simulink model "SPGF_FSK_0000_R2021b"  (R2021b)
settings: Solver=ode4  StartTime=0.0  StopTime=1.4  FixedStep=50e-6/50  RelTol=1e-3  EnableMultiTasking=on
undefined symbols (not defined in the file): D11, Delta
libraries: spsSeriesRLCBranchLib x1645, spsGroundLib x359, spsCurrentMeasurementLib x145, spsIdealSwitchLib x144, spsStairGeneratorLib x135, spsUniversalBridgeLib x76, spsThreePhaseSeriesRLCLoadLib x57, spsSequenceAnalyzerLib x31, simulink x24, spsThreePhaseParallelRLCLoadLib x20, spsThreePhaseTransformerTwoWindingsLib x20, spsDistributedParametersLineLib x19
(part 36 of 36)

== system SPGF_FSK_0000_R2021b/W51/Q/breaker ==
  Fault A2 : Constant  Value=InitialStatus(3)
  Fault A3 : Constant  Value=InitialStatus(2)
  Fault A4 : Constant  Value=InitialStatus(1)
  Fault C1 : Constant  Value=SwitchC
  Fault C2 : Constant  Value=SwitchB
  Fault C3 : Constant  Value=SwitchA
  Ideal Switch A : spsIdealSwitchLib/Ideal Switch  Ron=BreakerResistance  Lon=0  IC=InitialStatus(1)  Rs=SnubberResistance  Cs=SnubberCapacitance  Measurements=off
  Ideal Switch B : spsIdealSwitchLib/Ideal Switch  Ron=BreakerResistance  Lon=0  IC=InitialStatus(2)  Rs=SnubberResistance  Cs=SnubberCapacitance  Measurements=off
  Ideal Switch C : spsIdealSwitchLib/Ideal Switch  Ron=BreakerResistance  Lon=0  IC=InitialStatus(3)  Rs=SnubberResistance  Cs=SnubberCapacitance  Measurements=off
  Stair Generator A : spsStairGeneratorLib/Stair Generator  t=SwitchTimesA  e=SwitchStatusA  Ts=0
  Stair Generator B : spsStairGeneratorLib/Stair Generator  t=SwitchTimesB  e=SwitchStatusB  Ts=0
  Stair Generator C : spsStairGeneratorLib/Stair Generator  t=SwitchTimesC  e=SwitchStatusC  Ts=0
  Switch2 : Switch  Criteria=u2 > Threshold  Threshold=0.5
  Switch3 : Switch  Criteria=u2 > Threshold  Threshold=0.5
  Switch4 : Switch  Criteria=u2 > Threshold  Threshold=0.5
  A : PMIOPort  Side=Left
  B : PMIOPort  Port=2  Side=Left
  C : PMIOPort  Port=3  Side=Left
  a : PMIOPort  Port=4  Side=Right
  b : PMIOPort  Port=5  Side=Right
  c : PMIOPort  Port=6  Side=Right
  wires:
  Switch2/1 -> Ideal Switch C/1
  Fault A2/1 -> Switch2/3
  Fault C1/1 -> Switch2/2
  Switch3/1 -> Ideal Switch B/1
  Fault A3/1 -> Switch3/3
  Fault C2/1 -> Switch3/2
  Fault A4/1 -> Switch4/3
  Fault C3/1 -> Switch4/2
  Switch4/1 -> Ideal Switch A/1
  Stair Generator B/1 -> Switch3/1
  Stair Generator A/1 -> Switch4/1
  Stair Generator C/1 -> Switch2/1
  connections:
  Ideal Switch B/LConn1 -- B/RConn1
  Ideal Switch A/LConn1 -- A/RConn1
  Ideal Switch C/LConn1 -- C/RConn1
  Ideal Switch A/RConn1 -- a/RConn1
  b/RConn1 -- Ideal Switch B/RConn1
  c/RConn1 -- Ideal Switch C/RConn1

== system SPGF_FSK_0000_R2021b/W51/Q/meas ==
  Add : Sum  Inputs=+++
  GainI : Gain
  GainI0 : Gain
  I A: : spsCurrentMeasurementLib/Current Measurement  PhasorSimulation=off  OutputType=Complex  PSBequivalent=0
  I B: : spsCurrentMeasurementLib/Current Measurement  PhasorSimulation=off  OutputType=Complex  PSBequivalent=0
  I C: : spsCurrentMeasurementLib/Current Measurement  PhasorSimulation=off  OutputType=Complex  PSBequivalent=0
  Mux : Mux  Inputs=3
  A : PMIOPort  Side=Left
  B : PMIOPort  Port=2  Side=Left
  C : PMIOPort  Port=3  Side=Left
  a : PMIOPort  Port=4  Side=Right
  b : PMIOPort  Port=5  Side=Right
  c : PMIOPort  Port=6  Side=Right
  tag scope: CT3I0_W51=global, CTIabc_W51=global
  wires:
  I A:/1 -> Mux/1, Add/1
  I B:/1 -> Mux/2, Add/2
  I C:/1 -> Mux/3, Add/3
  Add/1 -> GainI0/1
  GainI0/1 -> [CT3I0_W51]
  Mux/1 -> GainI/1
  GainI/1 -> [CTIabc_W51]
  connections:
  I C:/RConn1 -- c/RConn1
  I B:/RConn1 -- b/RConn1
  a/RConn1 -- I A:/RConn1
  I A:/LConn1 -- A/RConn1
  I C:/LConn1 -- C/RConn1
  I B:/LConn1 -- B/RConn1

== system SPGF_FSK_0000_R2021b/W51/Q/shunt ==
  A : PMIOPort  Side=Left
  B : PMIOPort  Port=2  Side=Left
  C : PMIOPort  Port=3  Side=Left
  a : PMIOPort  Port=4  Side=Right
  b : PMIOPort  Port=5  Side=Right
  c : PMIOPort  Port=6  Side=Right
  connections:
  C/RConn1 -- c/RConn1
  B/RConn1 -- b/RConn1
  A/RConn1 -- a/RConn1

== system SPGF_FSK_0000_R2021b/W52/Q/breaker ==
  Fault A2 : Constant  Value=InitialStatus(3)
  Fault A3 : Constant  Value=InitialStatus(2)
  Fault A4 : Constant  Value=InitialStatus(1)
  Fault C1 : Constant  Value=SwitchC
  Fault C2 : Constant  Value=SwitchB
  Fault C3 : Constant  Value=SwitchA
  Ideal Switch A : spsIdealSwitchLib/Ideal Switch  Ron=BreakerResistance  Lon=0  IC=InitialStatus(1)  Rs=SnubberResistance  Cs=SnubberCapacitance  Measurements=off
  Ideal Switch B : spsIdealSwitchLib/Ideal Switch  Ron=BreakerResistance  Lon=0  IC=InitialStatus(2)  Rs=SnubberResistance  Cs=SnubberCapacitance  Measurements=off
  Ideal Switch C : spsIdealSwitchLib/Ideal Switch  Ron=BreakerResistance  Lon=0  IC=InitialStatus(3)  Rs=SnubberResistance  Cs=SnubberCapacitance  Measurements=off
  Stair Generator A : spsStairGeneratorLib/Stair Generator  t=SwitchTimesA  e=SwitchStatusA  Ts=0
  Stair Generator B : spsStairGeneratorLib/Stair Generator  t=SwitchTimesB  e=SwitchStatusB  Ts=0
  Stair Generator C : spsStairGeneratorLib/Stair Generator  t=SwitchTimesB  e=SwitchStatusB  Ts=0
  Switch2 : Switch  Criteria=u2 > Threshold  Threshold=0.5
  Switch3 : Switch  Criteria=u2 > Threshold  Threshold=0.5
  Switch4 : Switch  Criteria=u2 > Threshold  Threshold=0.5
  A : PMIOPort  Side=Left
  B : PMIOPort  Port=2  Side=Left
  C : PMIOPort  Port=3  Side=Left
  a : PMIOPort  Port=4  Side=Right
  b : PMIOPort  Port=5  Side=Right
  c : PMIOPort  Port=6  Side=Right
  wires:
  Switch2/1 -> Ideal Switch C/1
  Fault A2/1 -> Switch2/3
  Fault C1/1 -> Switch2/2
  Switch3/1 -> Ideal Switch B/1
  Fault A3/1 -> Switch3/3
  Fault C2/1 -> Switch3/2
  Fault A4/1 -> Switch4/3
  Fault C3/1 -> Switch4/2
  Switch4/1 -> Ideal Switch A/1
  Stair Generator B/1 -> Switch3/1
  Stair Generator A/1 -> Switch4/1
  Stair Generator C/1 -> Switch2/1
  connections:
  Ideal Switch B/LConn1 -- B/RConn1
  Ideal Switch A/LConn1 -- A/RConn1
  Ideal Switch C/LConn1 -- C/RConn1
  Ideal Switch A/RConn1 -- a/RConn1
  b/RConn1 -- Ideal Switch B/RConn1
  c/RConn1 -- Ideal Switch C/RConn1

== system SPGF_FSK_0000_R2021b/W52/Q/meas ==
  Add : Sum  Inputs=+++
  GainI : Gain
  GainI0 : Gain
  I A: : spsCurrentMeasurementLib/Current Measurement  PhasorSimulation=off  OutputType=Complex  PSBequivalent=0
  I B: : spsCurrentMeasurementLib/Current Measurement  PhasorSimulation=off  OutputType=Complex  PSBequivalent=0
  I C: : spsCurrentMeasurementLib/Current Measurement  PhasorSimulation=off  OutputType=Complex  PSBequivalent=0
  Mux : Mux  Inputs=3
  A : PMIOPort  Side=Left
  B : PMIOPort  Port=2  Side=Left
  C : PMIOPort  Port=3  Side=Left
  a : PMIOPort  Port=4  Side=Right
  b : PMIOPort  Port=5  Side=Right
  c : PMIOPort  Port=6  Side=Right
  tag scope: CT3I0_W52=global, CTIabc_W52=global
  wires:
  I A:/1 -> Mux/1, Add/1
  I B:/1 -> Mux/2, Add/2
  I C:/1 -> Mux/3, Add/3
  Add/1 -> GainI0/1
  GainI0/1 -> [CT3I0_W52]
  Mux/1 -> GainI/1
  GainI/1 -> [CTIabc_W52]
  connections:
  I C:/RConn1 -- c/RConn1
  I B:/RConn1 -- b/RConn1
  a/RConn1 -- I A:/RConn1
  I A:/LConn1 -- A/RConn1
  I C:/LConn1 -- C/RConn1
  I B:/LConn1 -- B/RConn1

== system SPGF_FSK_0000_R2021b/W52/Q/shunt ==
  A : PMIOPort  Side=Left
  B : PMIOPort  Port=2  Side=Left
  C : PMIOPort  Port=3  Side=Left
  a : PMIOPort  Port=4  Side=Right
  b : PMIOPort  Port=5  Side=Right
  c : PMIOPort  Port=6  Side=Right
  connections:
  C/RConn1 -- c/RConn1
  B/RConn1 -- b/RConn1
  A/RConn1 -- a/RConn1

== system SPGF_FSK_0000_R2021b/W53/Q/breaker ==
  Fault A2 : Constant  Value=InitialStatus(3)
  Fault A3 : Constant  Value=InitialStatus(2)
  Fault A4 : Constant  Value=InitialStatus(1)
  Fault C1 : Constant  Value=SwitchC
  Fault C2 : Constant  Value=SwitchB
  Fault C3 : Constant  Value=SwitchA
  Ideal Switch A : spsIdealSwitchLib/Ideal Switch  Ron=BreakerResistance  Lon=0  IC=InitialStatus(1)  Rs=SnubberResistance  Cs=SnubberCapacitance  Measurements=off
  Ideal Switch B : spsIdealSwitchLib/Ideal Switch  Ron=BreakerResistance  Lon=0  IC=InitialStatus(2)  Rs=SnubberResistance  Cs=SnubberCapacitance  Measurements=off
  Ideal Switch C : spsIdealSwitchLib/Ideal Switch  Ron=BreakerResistance  Lon=0  IC=InitialStatus(3)  Rs=SnubberResistance  Cs=SnubberCapacitance  Measurements=off
  Stair Generator A : spsStairGeneratorLib/Stair Generator  t=SwitchTimesA  e=SwitchStatusA  Ts=0
  Stair Generator B : spsStairGeneratorLib/Stair Generator  t=SwitchTimesB  e=SwitchStatusB  Ts=0
  Stair Generator C : spsStairGeneratorLib/Stair Generator  t=SwitchTimesB  e=SwitchStatusB  Ts=0
  Switch2 : Switch  Criteria=u2 > Threshold  Threshold=0.5
  Switch3 : Switch  Criteria=u2 > Threshold  Threshold=0.5
  Switch4 : Switch  Criteria=u2 > Threshold  Threshold=0.5
  A : PMIOPort  Side=Left
  B : PMIOPort  Port=2  Side=Left
  C : PMIOPort  Port=3  Side=Left
  a : PMIOPort  Port=4  Side=Right
  b : PMIOPort  Port=5  Side=Right
  c : PMIOPort  Port=6  Side=Right
  wires:
  Switch2/1 -> Ideal Switch C/1
  Fault A2/1 -> Switch2/3
  Fault C1/1 -> Switch2/2
  Switch3/1 -> Ideal Switch B/1
  Fault A3/1 -> Switch3/3
  Fault C2/1 -> Switch3/2
  Fault A4/1 -> Switch4/3
  Fault C3/1 -> Switch4/2
  Switch4/1 -> Ideal Switch A/1
  Stair Generator B/1 -> Switch3/1
  Stair Generator A/1 -> Switch4/1
  Stair Generator C/1 -> Switch2/1
  connections:
  Ideal Switch B/LConn1 -- B/RConn1
  Ideal Switch A/LConn1 -- A/RConn1
  Ideal Switch C/LConn1 -- C/RConn1
  Ideal Switch A/RConn1 -- a/RConn1
  b/RConn1 -- Ideal Switch B/RConn1
  c/RConn1 -- Ideal Switch C/RConn1

== system SPGF_FSK_0000_R2021b/W53/Q/meas ==
  Add : Sum  Inputs=+++
  GainI : Gain
  GainI0 : Gain
  I A: : spsCurrentMeasurementLib/Current Measurement  PhasorSimulation=off  OutputType=Complex  PSBequivalent=0
  I B: : spsCurrentMeasurementLib/Current Measurement  PhasorSimulation=off  OutputType=Complex  PSBequivalent=0
  I C: : spsCurrentMeasurementLib/Current Measurement  PhasorSimulation=off  OutputType=Complex  PSBequivalent=0
  Mux : Mux  Inputs=3
  A : PMIOPort  Side=Left
  B : PMIOPort  Port=2  Side=Left
  C : PMIOPort  Port=3  Side=Left
  a : PMIOPort  Port=4  Side=Right
  b : PMIOPort  Port=5  Side=Right
  c : PMIOPort  Port=6  Side=Right
  tag scope: CT3I0_W53=global, CTIabc_W53=global
  wires:
  I A:/1 -> Mux/1, Add/1
  I B:/1 -> Mux/2, Add/2
  I C:/1 -> Mux/3, Add/3
  Add/1 -> GainI0/1
  GainI0/1 -> [CT3I0_W53]
  Mux/1 -> GainI/1
  GainI/1 -> [CTIabc_W53]
  connections:
  I C:/RConn1 -- c/RConn1
  I B:/RConn1 -- b/RConn1
  a/RConn1 -- I A:/RConn1
  I A:/LConn1 -- A/RConn1
  I C:/LConn1 -- C/RConn1
  I B:/LConn1 -- B/RConn1

== system SPGF_FSK_0000_R2021b/W53/Q/shunt ==
  A : PMIOPort  Side=Left
  B : PMIOPort  Port=2  Side=Left
  C : PMIOPort  Port=3  Side=Left
  a : PMIOPort  Port=4  Side=Right
  b : PMIOPort  Port=5  Side=Right
  c : PMIOPort  Port=6  Side=Right
  connections:
  C/RConn1 -- c/RConn1
  B/RConn1 -- b/RConn1
  A/RConn1 -- a/RConn1

== system SPGF_FSK_0000_R2021b/W60/Q/breaker ==
  Fault A2 : Constant  Value=InitialStatus(3)
  Fault A3 : Constant  Value=InitialStatus(2)
  Fault A4 : Constant  Value=InitialStatus(1)
  Fault C1 : Constant  Value=SwitchC
  Fault C2 : Constant  Value=SwitchB
  Fault C3 : Constant  Value=SwitchA
  Ideal Switch A : spsIdealSwitchLib/Ideal Switch  Ron=BreakerResistance  Lon=0  IC=InitialStatus(1)  Rs=SnubberResistance  Cs=SnubberCapacitance  Measurements=off
  Ideal Switch B : spsIdealSwitchLib/Ideal Switch  Ron=BreakerResistance  Lon=0  IC=InitialStatus(2)  Rs=SnubberResistance  Cs=SnubberCapacitance  Measurements=off
  Ideal Switch C : spsIdealSwitchLib/Ideal Switch  Ron=BreakerResistance  Lon=0  IC=InitialStatus(3)  Rs=SnubberResistance  Cs=SnubberCapacitance  Measurements=off
  Stair Generator A : spsStairGeneratorLib/Stair Generator  t=SwitchTimesA  e=SwitchStatusA  Ts=0
  Stair Generator B : spsStairGeneratorLib/Stair Generator  t=SwitchTimesB  e=SwitchStatusB  Ts=0
  Stair Generator C : spsStairGeneratorLib/Stair Generator  t=SwitchTimesB  e=SwitchStatusB  Ts=0
  Switch2 : Switch  Criteria=u2 > Threshold  Threshold=0.5
  Switch3 : Switch  Criteria=u2 > Threshold  Threshold=0.5
  Switch4 : Switch  Criteria=u2 > Threshold  Threshold=0.5
  A : PMIOPort  Side=Left
  B : PMIOPort  Port=2  Side=Left
  C : PMIOPort  Port=3  Side=Left
  a : PMIOPort  Port=4  Side=Right
  b : PMIOPort  Port=5  Side=Right
  c : PMIOPort  Port=6  Side=Right
  wires:
  Switch2/1 -> Ideal Switch C/1
  Fault A2/1 -> Switch2/3
  Fault C1/1 -> Switch2/2
  Switch3/1 -> Ideal Switch B/1
  Fault A3/1 -> Switch3/3
  Fault C2/1 -> Switch3/2
  Fault A4/1 -> Switch4/3
  Fault C3/1 -> Switch4/2
  Switch4/1 -> Ideal Switch A/1
  Stair Generator B/1 -> Switch3/1
  Stair Generator A/1 -> Switch4/1
  Stair Generator C/1 -> Switch2/1
  connections:
  Ideal Switch B/LConn1 -- B/RConn1
  Ideal Switch A/LConn1 -- A/RConn1
  Ideal Switch C/LConn1 -- C/RConn1
  Ideal Switch A/RConn1 -- a/RConn1
  b/RConn1 -- Ideal Switch B/RConn1
  c/RConn1 -- Ideal Switch C/RConn1

== system SPGF_FSK_0000_R2021b/W60/Q/meas ==
  Add : Sum  Inputs=+++
  GainI : Gain
  GainI0 : Gain
  I A: : spsCurrentMeasurementLib/Current Measurement  PhasorSimulation=off  OutputType=Complex  PSBequivalent=0
  I B: : spsCurrentMeasurementLib/Current Measurement  PhasorSimulation=off  OutputType=Complex  PSBequivalent=0
  I C: : spsCurrentMeasurementLib/Current Measurement  PhasorSimulation=off  OutputType=Complex  PSBequivalent=0
  Mux : Mux  Inputs=3
  A : PMIOPort  Side=Left
  B : PMIOPort  Port=2  Side=Left
  C : PMIOPort  Port=3  Side=Left
  a : PMIOPort  Port=4  Side=Right
  b : PMIOPort  Port=5  Side=Right
  c : PMIOPort  Port=6  Side=Right
  tag scope: CT3I0_W60_1=global, CTIabc_W60_1=global
  wires:
  I A:/1 -> Mux/1, Add/1
  I B:/1 -> Mux/2, Add/2
  I C:/1 -> Mux/3, Add/3
  Add/1 -> GainI0/1
  GainI0/1 -> [CT3I0_W60_1]
  Mux/1 -> GainI/1
  GainI/1 -> [CTIabc_W60_1]
  connections:
  I C:/RConn1 -- c/RConn1
  I B:/RConn1 -- b/RConn1
  a/RConn1 -- I A:/RConn1
  I A:/LConn1 -- A/RConn1
  I C:/LConn1 -- C/RConn1
  I B:/LConn1 -- B/RConn1

== system SPGF_FSK_0000_R2021b/W60/Q/shunt ==
  A : PMIOPort  Side=Left
  B : PMIOPort  Port=2  Side=Left
  C : PMIOPort  Port=3  Side=Left
  a : PMIOPort  Port=4  Side=Right
  b : PMIOPort  Port=5  Side=Right
  c : PMIOPort  Port=6  Side=Right
  connections:
  C/RConn1 -- c/RConn1
  B/RConn1 -- b/RConn1
  A/RConn1 -- a/RConn1

== system SPGF_FSK_0000_R2021b/W61/Q/breaker ==
  Fault A2 : Constant  Value=InitialStatus(3)
  Fault A3 : Constant  Value=InitialStatus(2)
  Fault A4 : Constant  Value=InitialStatus(1)
  Fault C1 : Constant  Value=SwitchC
  Fault C2 : Constant  Value=SwitchB
  Fault C3 : Constant  Value=SwitchA
  Ideal Switch A : spsIdealSwitchLib/Ideal Switch  Ron=BreakerResistance  Lon=0  IC=InitialStatus(1)  Rs=SnubberResistance  Cs=SnubberCapacitance  Measurements=off
  Ideal Switch B : spsIdealSwitchLib/Ideal Switch  Ron=BreakerResistance  Lon=0  IC=InitialStatus(2)  Rs=SnubberResistance  Cs=SnubberCapacitance  Measurements=off
  Ideal Switch C : spsIdealSwitchLib/Ideal Switch  Ron=BreakerResistance  Lon=0  IC=InitialStatus(3)  Rs=SnubberResistance  Cs=SnubberCapacitance  Measurements=off
  Stair Generator A : spsStairGeneratorLib/Stair Generator  t=SwitchTimesA  e=SwitchStatusA  Ts=0
  Stair Generator B : spsStairGeneratorLib/Stair Generator  t=SwitchTimesB  e=SwitchStatusB  Ts=0
  Stair Generator C : spsStairGeneratorLib/Stair Generator  t=SwitchTimesB  e=SwitchStatusB  Ts=0
  Switch2 : Switch  Criteria=u2 > Threshold  Threshold=0.5
  Switch3 : Switch  Criteria=u2 > Threshold  Threshold=0.5
  Switch4 : Switch  Criteria=u2 > Threshold  Threshold=0.5
  A : PMIOPort  Side=Left
  B : PMIOPort  Port=2  Side=Left
  C : PMIOPort  Port=3  Side=Left
  a : PMIOPort  Port=4  Side=Right
  b : PMIOPort  Port=5  Side=Right
  c : PMIOPort  Port=6  Side=Right
  wires:
  Stair Generator C/1 -> Switch2/1
  Stair Generator A/1 -> Switch4/1
  Stair Generator B/1 -> Switch3/1
  Switch4/1 -> Ideal Switch A/1
  Fault C3/1 -> Switch4/2
  Fault A4/1 -> Switch4/3
  Fault C2/1 -> Switch3/2
  Fault A3/1 -> Switch3/3
  Switch3/1 -> Ideal Switch B/1
  Fault C1/1 -> Switch2/2
  Fault A2/1 -> Switch2/3
  Switch2/1 -> Ideal Switch C/1
  connections:
  c/RConn1 -- Ideal Switch C/RConn1
  b/RConn1 -- Ideal Switch B/RConn1
  Ideal Switch A/RConn1 -- a/RConn1
  Ideal Switch C/LConn1 -- C/RConn1
  Ideal Switch A/LConn1 -- A/RConn1
  Ideal Switch B/LConn1 -- B/RConn1

== system SPGF_FSK_0000_R2021b/W61/Q/meas ==
  Add : Sum  Inputs=+++
  GainI : Gain
  GainI0 : Gain
  I A: : spsCurrentMeasurementLib/Current Measurement  PhasorSimulation=off  OutputType=Complex  PSBequivalent=0
  I B: : spsCurrentMeasurementLib/Current Measurement  PhasorSimulation=off  OutputType=Complex  PSBequivalent=0
  I C: : spsCurrentMeasurementLib/Current Measurement  PhasorSimulation=off  OutputType=Complex  PSBequivalent=0
  Mux : Mux  Inputs=3
  A : PMIOPort  Side=Left
  B : PMIOPort  Port=2  Side=Left
  C : PMIOPort  Port=3  Side=Left
  a : PMIOPort  Port=4  Side=Right
  b : PMIOPort  Port=5  Side=Right
  c : PMIOPort  Port=6  Side=Right
  tag scope: CT3I0_W60_2=global, CTIabc_W60_2=global
  wires:
  GainI/1 -> [CTIabc_W60_2]
  Mux/1 -> GainI/1
  GainI0/1 -> [CT3I0_W60_2]
  Add/1 -> GainI0/1
  I C:/1 -> Add/3, Mux/3
  I B:/1 -> Add/2, Mux/2
  I A:/1 -> Add/1, Mux/1
  connections:
  I B:/LConn1 -- B/RConn1
  I C:/LConn1 -- C/RConn1
  I A:/LConn1 -- A/RConn1
  a/RConn1 -- I A:/RConn1
  I B:/RConn1 -- b/RConn1
  I C:/RConn1 -- c/RConn1

== system SPGF_FSK_0000_R2021b/W61/Q/shunt ==
  A : PMIOPort  Side=Left
  B : PMIOPort  Port=2  Side=Left
  C : PMIOPort  Port=3  Side=Left
  a : PMIOPort  Port=4  Side=Right
  b : PMIOPort  Port=5  Side=Right
  c : PMIOPort  Port=6  Side=Right
  connections:
  A/RConn1 -- a/RConn1
  B/RConn1 -- b/RConn1
  C/RConn1 -- c/RConn1

== system SPGF_FSK_0000_R2021b/K1/fault/Arcing/R-S Flip-Flop ==
  S : Inport
  R : Inport  Port=2
  Demux2 : Demux  Outputs=2
      settings: DisplayOption=none
  Logic : CombinatorialLogic  TruthTable=[0 1;1 0;0 1;0 1;1 0;1 0;1 1;1 1]
  Memory : Memory  InitialCondition=InitialCondition  InheritSampleTime=on
  Mux2 : Mux  Inputs=3
  Q : Outport  InitialOutput=0
  !Q : Outport  Port=2  InitialOutput=1
  wires:
  S/1 -> Mux2/1
  Demux2/2 -> !Q/1
  Mux2/1 -> Logic/1
  Demux2/1 -> Q/1, Memory/1
  Logic/1 -> Demux2/1
  Memory/1 -> Mux2/3
  R/1 -> Mux2/2

== system SPGF_FSK_0000_R2021b/K1/fault/Arcing/Triggered Subsystem1 ==
  I : Inport
  Trigger : TriggerPort  VariantControl=Variant
  O : Outport
  wires:
  I/1 -> O/1

== system SPGF_FSK_0000_R2021b/K1/fault/Count Limiter/Counter ==
  I : Inport
  Trigger : TriggerPort  TriggerType=falling  VariantControl=Variant
  Add : Sum
  Memory : Memory  InheritSampleTime=on
  O : Outport
  wires:
  Add/1 -> O/1, Memory/1
  Memory/1 -> Add/2
  I/1 -> Add/1

== system SPGF_FSK_0000_R2021b/K1/fault/Time Delay/SC_Time5 ==
  Control : Inport
  TimeDelay : Inport  Port=2
  Clock1 : Clock
  Memory : Memory
  Product : Product  RndMeth=Zero
  Triggered Subsystem1 : Subsystem  TreatAsAtomicUnit=on
  Out : Outport
  wires:
  Triggered Subsystem1/1(Out) -> Product/2
  Clock1/1 -> Triggered Subsystem1/3(Clock)
  TimeDelay/1 -> Triggered Subsystem1/2(Time)
  Control/1 -> Triggered Subsystem1/1(Tr), Product/1, Triggered Subsystem1/Enable
  Product/1 -> Memory/1
  Memory/1 -> Out/1

== system SPGF_FSK_0000_R2021b/K2/fault/Arcing/R-S Flip-Flop ==
  S : Inport
  R : Inport  Port=2
  Demux2 : Demux  Outputs=2
      settings: DisplayOption=none
  Logic : CombinatorialLogic  TruthTable=[0 1;1 0;0 1;0 1;1 0;1 0;1 1;1 1]
  Memory : Memory  InitialCondition=InitialCondition  InheritSampleTime=on
  Mux2 : Mux  Inputs=3
  Q : Outport  InitialOutput=0
  !Q : Outport  Port=2  InitialOutput=1
  wires:
  S/1 -> Mux2/1
  Demux2/2 -> !Q/1
  Mux2/1 -> Logic/1
  Demux2/1 -> Q/1, Memory/1
  Logic/1 -> Demux2/1
  Memory/1 -> Mux2/3
  R/1 -> Mux2/2

== system SPGF_FSK_0000_R2021b/K2/fault/Arcing/Triggered Subsystem1 ==
  I : Inport
  Trigger : TriggerPort  VariantControl=Variant
  O : Outport
  wires:
  I/1 -> O/1

== system SPGF_FSK_0000_R2021b/K2/fault/Count Limiter/Counter ==
  I : Inport
  Trigger : TriggerPort  TriggerType=falling  VariantControl=Variant
  Add : Sum
  Memory : Memory  InheritSampleTime=on
  O : Outport
  wires:
  Add/1 -> O/1, Memory/1
  Memory/1 -> Add/2
  I/1 -> Add/1

== system SPGF_FSK_0000_R2021b/K2/fault/Time Delay/SC_Time5 ==
  Control : Inport
  TimeDelay : Inport  Port=2
  Clock1 : Clock
  Memory : Memory
  Product : Product  RndMeth=Zero
  Triggered Subsystem1 : Subsystem  TreatAsAtomicUnit=on
  Out : Outport
  wires:
  Triggered Subsystem1/1(Out) -> Product/2
  Clock1/1 -> Triggered Subsystem1/3(Clock)
  TimeDelay/1 -> Triggered Subsystem1/2(Time)
  Control/1 -> Triggered Subsystem1/1(Tr), Product/1, Triggered Subsystem1/Enable
  Product/1 -> Memory/1
  Memory/1 -> Out/1

== system SPGF_FSK_0000_R2021b/K3/fault/Arcing/R-S Flip-Flop ==
  S : Inport
  R : Inport  Port=2
  Demux2 : Demux  Outputs=2
      settings: DisplayOption=none
  Logic : CombinatorialLogic  TruthTable=[0 1;1 0;0 1;0 1;1 0;1 0;1 1;1 1]
  Memory : Memory  InitialCondition=InitialCondition  InheritSampleTime=on
  Mux2 : Mux  Inputs=3
  Q : Outport  InitialOutput=0
  !Q : Outport  Port=2  InitialOutput=1
  wires:
  S/1 -> Mux2/1
  Demux2/2 -> !Q/1
  Mux2/1 -> Logic/1
  Demux2/1 -> Q/1, Memory/1
  Logic/1 -> Demux2/1
  Memory/1 -> Mux2/3
  R/1 -> Mux2/2

== system SPGF_FSK_0000_R2021b/K3/fault/Arcing/Triggered Subsystem1 ==
  I : Inport
  Trigger : TriggerPort  VariantControl=Variant
  O : Outport
  wires:
  I/1 -> O/1

== system SPGF_FSK_0000_R2021b/K3/fault/Count Limiter/Counter ==
  I : Inport
  Trigger : TriggerPort  TriggerType=falling  VariantControl=Variant
  Add : Sum
  Memory : Memory  InheritSampleTime=on
  O : Outport
  wires:
  Add/1 -> O/1, Memory/1
  Memory/1 -> Add/2
  I/1 -> Add/1

== system SPGF_FSK_0000_R2021b/K3/fault/Time Delay/SC_Time5 ==
  Control : Inport
  TimeDelay : Inport  Port=2
  Clock1 : Clock
  Memory : Memory
  Product : Product  RndMeth=Zero
  Triggered Subsystem1 : Subsystem  TreatAsAtomicUnit=on
  Out : Outport
  wires:
  Triggered Subsystem1/1(Out) -> Product/2
  Clock1/1 -> Triggered Subsystem1/3(Clock)
  TimeDelay/1 -> Triggered Subsystem1/2(Time)
  Control/1 -> Triggered Subsystem1/1(Tr), Product/1, Triggered Subsystem1/Enable
  Product/1 -> Memory/1
  Memory/1 -> Out/1

== system SPGF_FSK_0000_R2021b/K4/fault/Arcing/R-S Flip-Flop ==
  S : Inport
  R : Inport  Port=2
  Demux2 : Demux  Outputs=2
      settings: DisplayOption=none
  Logic : CombinatorialLogic  TruthTable=[0 1;1 0;0 1;0 1;1 0;1 0;1 1;1 1]
  Memory : Memory  InitialCondition=InitialCondition  InheritSampleTime=on
  Mux2 : Mux  Inputs=3
  Q : Outport  InitialOutput=0
  !Q : Outport  Port=2  InitialOutput=1
  wires:
  S/1 -> Mux2/1
  Demux2/2 -> !Q/1
  Mux2/1 -> Logic/1
  Demux2/1 -> Q/1, Memory/1
  Logic/1 -> Demux2/1
  Memory/1 -> Mux2/3
  R/1 -> Mux2/2

== system SPGF_FSK_0000_R2021b/K4/fault/Arcing/Triggered Subsystem1 ==
  I : Inport
  Trigger : TriggerPort  VariantControl=Variant
  O : Outport
  wires:
  I/1 -> O/1

== system SPGF_FSK_0000_R2021b/K4/fault/Count Limiter/Counter ==
  I : Inport
  Trigger : TriggerPort  TriggerType=falling  VariantControl=Variant
  Add : Sum
  Memory : Memory  InheritSampleTime=on
  O : Outport
  wires:
  Add/1 -> O/1, Memory/1
  Memory/1 -> Add/2
  I/1 -> Add/1

== system SPGF_FSK_0000_R2021b/K4/fault/Time Delay/SC_Time5 ==
  Control : Inport
  TimeDelay : Inport  Port=2
  Clock1 : Clock
  Memory : Memory
  Product : Product  RndMeth=Zero
  Triggered Subsystem1 : Subsystem  TreatAsAtomicUnit=on
  Out : Outport
  wires:
  Triggered Subsystem1/1(Out) -> Product/2
  Clock1/1 -> Triggered Subsystem1/3(Clock)
  TimeDelay/1 -> Triggered Subsystem1/2(Time)
  Control/1 -> Triggered Subsystem1/1(Tr), Product/1, Triggered Subsystem1/Enable
  Product/1 -> Memory/1
  Memory/1 -> Out/1

== system SPGF_FSK_0000_R2021b/K5/fault/Arcing/R-S Flip-Flop ==
  S : Inport
  R : Inport  Port=2
  Demux2 : Demux  Outputs=2
      settings: DisplayOption=none
  Logic : CombinatorialLogic  TruthTable=[0 1;1 0;0 1;0 1;1 0;1 0;1 1;1 1]
  Memory : Memory  InitialCondition=InitialCondition  InheritSampleTime=on
  Mux2 : Mux  Inputs=3
  Q : Outport  InitialOutput=0
  !Q : Outport  Port=2  InitialOutput=1
  wires:
  S/1 -> Mux2/1
  Demux2/2 -> !Q/1
  Mux2/1 -> Logic/1
  Demux2/1 -> Q/1, Memory/1
  Logic/1 -> Demux2/1
  Memory/1 -> Mux2/3
  R/1 -> Mux2/2

== system SPGF_FSK_0000_R2021b/K5/fault/Arcing/Triggered Subsystem1 ==
  I : Inport
  Trigger : TriggerPort  VariantControl=Variant
  O : Outport
  wires:
  I/1 -> O/1

== system SPGF_FSK_0000_R2021b/K5/fault/Count Limiter/Counter ==
  I : Inport
  Trigger : TriggerPort  TriggerType=falling  VariantControl=Variant
  Add : Sum
  Memory : Memory  InheritSampleTime=on
  O : Outport
  wires:
  Add/1 -> O/1, Memory/1
  Memory/1 -> Add/2
  I/1 -> Add/1

== system SPGF_FSK_0000_R2021b/K5/fault/Time Delay/SC_Time5 ==
  Control : Inport
  TimeDelay : Inport  Port=2
  Clock1 : Clock
  Memory : Memory
  Product : Product  RndMeth=Zero
  Triggered Subsystem1 : Subsystem  TreatAsAtomicUnit=on
  Out : Outport
  wires:
  Triggered Subsystem1/1(Out) -> Product/2
  Clock1/1 -> Triggered Subsystem1/3(Clock)
  TimeDelay/1 -> Triggered Subsystem1/2(Time)
  Control/1 -> Triggered Subsystem1/1(Tr), Product/1, Triggered Subsystem1/Enable
  Product/1 -> Memory/1
  Memory/1 -> Out/1

== system SPGF_FSK_0000_R2021b/K6/fault/Arcing/R-S Flip-Flop ==
  S : Inport
  R : Inport  Port=2
  Demux2 : Demux  Outputs=2
      settings: DisplayOption=none
  Logic : CombinatorialLogic  TruthTable=[0 1;1 0;0 1;0 1;1 0;1 0;1 1;1 1]
  Memory : Memory  InitialCondition=InitialCondition  InheritSampleTime=on
  Mux2 : Mux  Inputs=3
  Q : Outport  InitialOutput=0
  !Q : Outport  Port=2  InitialOutput=1
  wires:
  S/1 -> Mux2/1
  Demux2/2 -> !Q/1
  Mux2/1 -> Logic/1
  Demux2/1 -> Q/1, Memory/1
  Logic/1 -> Demux2/1
  Memory/1 -> Mux2/3
  R/1 -> Mux2/2

== system SPGF_FSK_0000_R2021b/K6/fault/Arcing/Triggered Subsystem1 ==
  I : Inport
  Trigger : TriggerPort  VariantControl=Variant
  O : Outport
  wires:
  I/1 -> O/1

== system SPGF_FSK_0000_R2021b/K6/fault/Count Limiter/Counter ==
  I : Inport
  Trigger : TriggerPort  TriggerType=falling  VariantControl=Variant
  Add : Sum
  Memory : Memory  InheritSampleTime=on
  O : Outport
  wires:
  Add/1 -> O/1, Memory/1
  Memory/1 -> Add/2
  I/1 -> Add/1

== system SPGF_FSK_0000_R2021b/K6/fault/Time Delay/SC_Time5 ==
  Control : Inport
  TimeDelay : Inport  Port=2
  Clock1 : Clock
  Memory : Memory
  Product : Product  RndMeth=Zero
  Triggered Subsystem1 : Subsystem  TreatAsAtomicUnit=on
  Out : Outport
  wires:
  Triggered Subsystem1/1(Out) -> Product/2
  Clock1/1 -> Triggered Subsystem1/3(Clock)
  TimeDelay/1 -> Triggered Subsystem1/2(Time)
  Control/1 -> Triggered Subsystem1/1(Tr), Product/1, Triggered Subsystem1/Enable
  Product/1 -> Memory/1
  Memory/1 -> Out/1

== system SPGF_FSK_0000_R2021b/K8/fault/Arcing/R-S Flip-Flop ==
  S : Inport
  R : Inport  Port=2
  Demux2 : Demux  Outputs=2
      settings: DisplayOption=none
  Logic : CombinatorialLogic  TruthTable=[0 1;1 0;0 1;0 1;1 0;1 0;1 1;1 1]
  Memory : Memory  InitialCondition=InitialCondition  InheritSampleTime=on
  Mux2 : Mux  Inputs=3
  Q : Outport  InitialOutput=0
  !Q : Outport  Port=2  InitialOutput=1
  wires:
  R/1 -> Mux2/2
  Memory/1 -> Mux2/3
  Logic/1 -> Demux2/1
  Demux2/1 -> Memory/1, Q/1
  Mux2/1 -> Logic/1
  Demux2/2 -> !Q/1
  S/1 -> Mux2/1

== system SPGF_FSK_0000_R2021b/K8/fault/Arcing/Triggered Subsystem1 ==
  I : Inport
  Trigger : TriggerPort  VariantControl=Variant
  O : Outport
  wires:
  I/1 -> O/1

== system SPGF_FSK_0000_R2021b/K8/fault/Count Limiter/Counter ==
  I : Inport
  Trigger : TriggerPort  TriggerType=falling  VariantControl=Variant
  Add : Sum
  Memory : Memory  InheritSampleTime=on
  O : Outport
  wires:
  I/1 -> Add/1
  Memory/1 -> Add/2
  Add/1 -> Memory/1, O/1

== system SPGF_FSK_0000_R2021b/K8/fault/Time Delay/SC_Time5 ==
  Control : Inport
  TimeDelay : Inport  Port=2
  Clock1 : Clock
  Memory : Memory
  Product : Product  RndMeth=Zero
  Triggered Subsystem1 : Subsystem  TreatAsAtomicUnit=on
  Out : Outport
  wires:
  Memory/1 -> Out/1
  Product/1 -> Memory/1
  Control/1 -> Triggered Subsystem1/Enable, Product/1, Triggered Subsystem1/1(Tr)
  TimeDelay/1 -> Triggered Subsystem1/2(Time)
  Clock1/1 -> Triggered Subsystem1/3(Clock)
  Triggered Subsystem1/1(Out) -> Product/2

== system SPGF_FSK_0000_R2021b/K9/fault/Arcing/R-S Flip-Flop ==
  S : Inport
  R : Inport  Port=2
  Demux2 : Demux  Outputs=2
      settings: DisplayOption=none
  Logic : CombinatorialLogic  TruthTable=[0 1;1 0;0 1;0 1;1 0;1 0;1 1;1 1]
  Memory : Memory  InitialCondition=InitialCondition  InheritSampleTime=on
  Mux2 : Mux  Inputs=3
  Q : Outport  InitialOutput=0
  !Q : Outport  Port=2  InitialOutput=1
  wires:
  S/1 -> Mux2/1
  Demux2/2 -> !Q/1
  Mux2/1 -> Logic/1
  Demux2/1 -> Q/1, Memory/1
  Logic/1 -> Demux2/1
  Memory/1 -> Mux2/3
  R/1 -> Mux2/2

== system SPGF_FSK_0000_R2021b/K9/fault/Arcing/Triggered Subsystem1 ==
  I : Inport
  Trigger : TriggerPort  VariantControl=Variant
  O : Outport
  wires:
  I/1 -> O/1

== system SPGF_FSK_0000_R2021b/K9/fault/Count Limiter/Counter ==
  I : Inport
  Trigger : TriggerPort  TriggerType=falling  VariantControl=Variant
  Add : Sum
  Memory : Memory  InheritSampleTime=on
  O : Outport
  wires:
  Add/1 -> O/1, Memory/1
  Memory/1 -> Add/2
  I/1 -> Add/1

== system SPGF_FSK_0000_R2021b/K9/fault/Time Delay/SC_Time5 ==
  Control : Inport
  TimeDelay : Inport  Port=2
  Clock1 : Clock
  Memory : Memory
  Product : Product  RndMeth=Zero
  Triggered Subsystem1 : Subsystem  TreatAsAtomicUnit=on
  Out : Outport
  wires:
  Triggered Subsystem1/1(Out) -> Product/2
  Clock1/1 -> Triggered Subsystem1/3(Clock)
  TimeDelay/1 -> Triggered Subsystem1/2(Time)
  Control/1 -> Triggered Subsystem1/1(Tr), Product/1, Triggered Subsystem1/Enable
  Product/1 -> Memory/1
  Memory/1 -> Out/1

== system SPGF_FSK_0000_R2021b/K1/fault/Time Delay/SC_Time5/Triggered Subsystem1 ==
  Tr : Inport
  Time : Inport  Port=2
  Clock : Inport  Port=3
  Enable : EnablePort
  Add : Sum
  Memory3 : Memory  InheritSampleTime=on
  Memory4 : Memory  InheritSampleTime=on
  Relational Operator : RelationalOperator  Operator=>  OutDataTypeStr=boolean  RndMeth=Nearest
  Triggered Subsystem2 : Subsystem  TreatAsAtomicUnit=on
  Out : Outport  InitialOutput=0
  wires:
  Memory4/1 -> Triggered Subsystem2/Trigger
  Memory3/1 -> Relational Operator/1
  Clock/1 -> Triggered Subsystem2/1(In1), Memory3/1
  Relational Operator/1 -> Out/1
  Time/1 -> Add/2
  Tr/1 -> Memory4/1
  Add/1 -> Relational Operator/2
  Triggered Subsystem2/1(Out1) -> Add/1

== system SPGF_FSK_0000_R2021b/K2/fault/Time Delay/SC_Time5/Triggered Subsystem1 ==
  Tr : Inport
  Time : Inport  Port=2
  Clock : Inport  Port=3
  Enable : EnablePort
  Add : Sum
  Memory3 : Memory  InheritSampleTime=on
  Memory4 : Memory  InheritSampleTime=on
  Relational Operator : RelationalOperator  Operator=>  OutDataTypeStr=boolean  RndMeth=Nearest
  Triggered Subsystem2 : Subsystem  TreatAsAtomicUnit=on
  Out : Outport  InitialOutput=0
  wires:
  Memory4/1 -> Triggered Subsystem2/Trigger
  Memory3/1 -> Relational Operator/1
  Clock/1 -> Triggered Subsystem2/1(In1), Memory3/1
  Relational Operator/1 -> Out/1
  Time/1 -> Add/2
  Tr/1 -> Memory4/1
  Add/1 -> Relational Operator/2
  Triggered Subsystem2/1(Out1) -> Add/1

== system SPGF_FSK_0000_R2021b/K3/fault/Time Delay/SC_Time5/Triggered Subsystem1 ==
  Tr : Inport
  Time : Inport  Port=2
  Clock : Inport  Port=3
  Enable : EnablePort
  Add : Sum
  Memory3 : Memory  InheritSampleTime=on
  Memory4 : Memory  InheritSampleTime=on
  Relational Operator : RelationalOperator  Operator=>  OutDataTypeStr=boolean  RndMeth=Nearest
  Triggered Subsystem2 : Subsystem  TreatAsAtomicUnit=on
  Out : Outport  InitialOutput=0
  wires:
  Memory4/1 -> Triggered Subsystem2/Trigger
  Memory3/1 -> Relational Operator/1
  Clock/1 -> Triggered Subsystem2/1(In1), Memory3/1
  Relational Operator/1 -> Out/1
  Time/1 -> Add/2
  Tr/1 -> Memory4/1
  Add/1 -> Relational Operator/2
  Triggered Subsystem2/1(Out1) -> Add/1

== system SPGF_FSK_0000_R2021b/K4/fault/Time Delay/SC_Time5/Triggered Subsystem1 ==
  Tr : Inport
  Time : Inport  Port=2
  Clock : Inport  Port=3
  Enable : EnablePort
  Add : Sum
  Memory3 : Memory  InheritSampleTime=on
  Memory4 : Memory  InheritSampleTime=on
  Relational Operator : RelationalOperator  Operator=>  OutDataTypeStr=boolean  RndMeth=Nearest
  Triggered Subsystem2 : Subsystem  TreatAsAtomicUnit=on
  Out : Outport  InitialOutput=0
  wires:
  Memory4/1 -> Triggered Subsystem2/Trigger
  Memory3/1 -> Relational Operator/1
  Clock/1 -> Triggered Subsystem2/1(In1), Memory3/1
  Relational Operator/1 -> Out/1
  Time/1 -> Add/2
  Tr/1 -> Memory4/1
  Add/1 -> Relational Operator/2
  Triggered Subsystem2/1(Out1) -> Add/1

== system SPGF_FSK_0000_R2021b/K5/fault/Time Delay/SC_Time5/Triggered Subsystem1 ==
  Tr : Inport
  Time : Inport  Port=2
  Clock : Inport  Port=3
  Enable : EnablePort
  Add : Sum
  Memory3 : Memory  InheritSampleTime=on
  Memory4 : Memory  InheritSampleTime=on
  Relational Operator : RelationalOperator  Operator=>  OutDataTypeStr=boolean  RndMeth=Nearest
  Triggered Subsystem2 : Subsystem  TreatAsAtomicUnit=on
  Out : Outport  InitialOutput=0
  wires:
  Memory4/1 -> Triggered Subsystem2/Trigger
  Memory3/1 -> Relational Operator/1
  Clock/1 -> Triggered Subsystem2/1(In1), Memory3/1
  Relational Operator/1 -> Out/1
  Time/1 -> Add/2
  Tr/1 -> Memory4/1
  Add/1 -> Relational Operator/2
  Triggered Subsystem2/1(Out1) -> Add/1

== system SPGF_FSK_0000_R2021b/K6/fault/Time Delay/SC_Time5/Triggered Subsystem1 ==
  Tr : Inport
  Time : Inport  Port=2
  Clock : Inport  Port=3
  Enable : EnablePort
  Add : Sum
  Memory3 : Memory  InheritSampleTime=on
  Memory4 : Memory  InheritSampleTime=on
  Relational Operator : RelationalOperator  Operator=>  OutDataTypeStr=boolean  RndMeth=Nearest
  Triggered Subsystem2 : Subsystem  TreatAsAtomicUnit=on
  Out : Outport  InitialOutput=0
  wires:
  Memory4/1 -> Triggered Subsystem2/Trigger
  Memory3/1 -> Relational Operator/1
  Clock/1 -> Triggered Subsystem2/1(In1), Memory3/1
  Relational Operator/1 -> Out/1
  Time/1 -> Add/2
  Tr/1 -> Memory4/1
  Add/1 -> Relational Operator/2
  Triggered Subsystem2/1(Out1) -> Add/1

== system SPGF_FSK_0000_R2021b/K8/fault/Time Delay/SC_Time5/Triggered Subsystem1 ==
  Tr : Inport
  Time : Inport  Port=2
  Clock : Inport  Port=3
  Enable : EnablePort
  Add : Sum
  Memory3 : Memory  InheritSampleTime=on
  Memory4 : Memory  InheritSampleTime=on
  Relational Operator : RelationalOperator  Operator=>  OutDataTypeStr=boolean  RndMeth=Nearest
  Triggered Subsystem2 : Subsystem  TreatAsAtomicUnit=on
  Out : Outport  InitialOutput=0
  wires:
  Triggered Subsystem2/1(Out1) -> Add/1
  Add/1 -> Relational Operator/2
  Tr/1 -> Memory4/1
  Time/1 -> Add/2
  Relational Operator/1 -> Out/1
  Clock/1 -> Memory3/1, Triggered Subsystem2/1(In1)
  Memory3/1 -> Relational Operator/1
  Memory4/1 -> Triggered Subsystem2/Trigger

== system SPGF_FSK_0000_R2021b/K9/fault/Time Delay/SC_Time5/Triggered Subsystem1 ==
  Tr : Inport
  Time : Inport  Port=2
  Clock : Inport  Port=3
  Enable : EnablePort
  Add : Sum
  Memory3 : Memory  InheritSampleTime=on
  Memory4 : Memory  InheritSampleTime=on
  Relational Operator : RelationalOperator  Operator=>  OutDataTypeStr=boolean  RndMeth=Nearest
  Triggered Subsystem2 : Subsystem  TreatAsAtomicUnit=on
  Out : Outport  InitialOutput=0
  wires:
  Memory4/1 -> Triggered Subsystem2/Trigger
  Memory3/1 -> Relational Operator/1
  Clock/1 -> Triggered Subsystem2/1(In1), Memory3/1
  Relational Operator/1 -> Out/1
  Time/1 -> Add/2
  Tr/1 -> Memory4/1
  Add/1 -> Relational Operator/2
  Triggered Subsystem2/1(Out1) -> Add/1

== system SPGF_FSK_0000_R2021b/K1/fault/Time Delay/SC_Time5/Triggered Subsystem1/Triggered Subsystem2 ==
  In1 : Inport
  Trigger : TriggerPort  VariantControl=Variant
  Out1 : Outport  InitialOutput=0
  wires:
  In1/1 -> Out1/1

== system SPGF_FSK_0000_R2021b/K2/fault/Time Delay/SC_Time5/Triggered Subsystem1/Triggered Subsystem2 ==
  In1 : Inport
  Trigger : TriggerPort  VariantControl=Variant
  Out1 : Outport  InitialOutput=0
  wires:
  In1/1 -> Out1/1

== system SPGF_FSK_0000_R2021b/K3/fault/Time Delay/SC_Time5/Triggered Subsystem1/Triggered Subsystem2 ==
  In1 : Inport
  Trigger : TriggerPort  VariantControl=Variant
  Out1 : Outport  InitialOutput=0
  wires:
  In1/1 -> Out1/1

== system SPGF_FSK_0000_R2021b/K4/fault/Time Delay/SC_Time5/Triggered Subsystem1/Triggered Subsystem2 ==
  In1 : Inport
  Trigger : TriggerPort  VariantControl=Variant
  Out1 : Outport  InitialOutput=0
  wires:
  In1/1 -> Out1/1

== system SPGF_FSK_0000_R2021b/K5/fault/Time Delay/SC_Time5/Triggered Subsystem1/Triggered Subsystem2 ==
  In1 : Inport
  Trigger : TriggerPort  VariantControl=Variant
  Out1 : Outport  InitialOutput=0
  wires:
  In1/1 -> Out1/1

== system SPGF_FSK_0000_R2021b/K6/fault/Time Delay/SC_Time5/Triggered Subsystem1/Triggered Subsystem2 ==
  In1 : Inport
  Trigger : TriggerPort  VariantControl=Variant
  Out1 : Outport  InitialOutput=0
  wires:
  In1/1 -> Out1/1

== system SPGF_FSK_0000_R2021b/K8/fault/Time Delay/SC_Time5/Triggered Subsystem1/Triggered Subsystem2 ==
  In1 : Inport
  Trigger : TriggerPort  VariantControl=Variant
  Out1 : Outport  InitialOutput=0
  wires:
  In1/1 -> Out1/1

== system SPGF_FSK_0000_R2021b/K9/fault/Time Delay/SC_Time5/Triggered Subsystem1/Triggered Subsystem2 ==
  In1 : Inport
  Trigger : TriggerPort  VariantControl=Variant
  Out1 : Outport  InitialOutput=0
  wires:
  In1/1 -> Out1/1
